simulink model "P8_simulink"  (R2023b)
settings: Solver=VariableStepAuto  StartTime=0.0  StopTime=10.0  RelTol=1e-3
values from neighbouring files (symbols this model uses):
  b = 0.0012    [P8_SisElecMec.m]    (also in P8_parameters.mat)
  J = 0.001    [P8_SisElecMec.m]    (also in P8_parameters.mat)
  Ke = 0.01    [P8_parameters.mat]
  Kt = 0.01    [P8_parameters.mat]
  La = 0.023    [P8_parameters.mat]
  Ra = 2    [P8_parameters.mat]
  T = 0    [P8_SisElecMec.m]    (also in P8_parameters.mat)

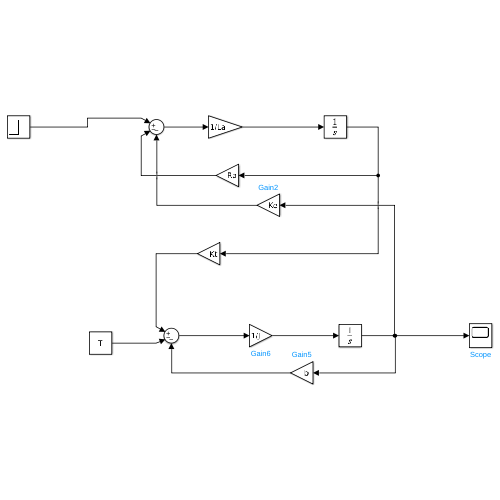
[thumbnail: Simulink's stored preview of the top-level diagram]
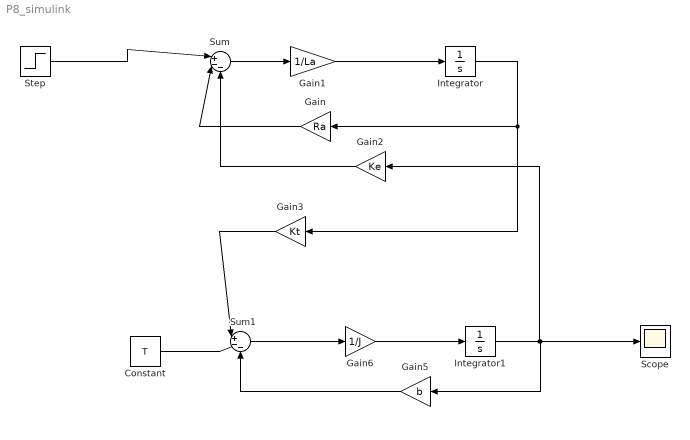
== system P8_simulink ==
  Constant : Constant  Value=T
  Gain : Gain  Gain=Ra
  Gain1 : Gain  Gain=1/La
  Gain2 : Gain  Gain=Ke
  Gain3 : Gain  Gain=Kt
  Gain5 : Gain  Gain=b
  Gain6 : Gain  Gain=1/J
  Integrator : Integrator
  Integrator1 : Integrator
  Scope : Scope
  Step : Step  Time=0  After=5  SampleTime=0
  Sum : Sum  Inputs=|+--
  Sum1 : Sum  Inputs=|+--
  wires:
  Step/1 -> Sum/1
  Sum/1 -> Gain1/1
  Gain1/1 -> Integrator/1
  Integrator/1 -> Gain3/1, Gain/1
  Gain/1 -> Sum/2
  Gain2/1 -> Sum/3
  Gain6/1 -> Integrator1/1
  Sum1/1 -> Gain6/1
  Integrator1/1 -> Scope/1, Gain5/1, Gain2/1
  Gain3/1 -> Sum1/1
  Constant/1 -> Sum1/2
  Gain5/1 -> Sum1/3
